simulink model "Laboratoria_nr_6_filtr_SIMULINK"  (R2019a)
settings: Solver=VariableStepAuto  StartTime=0.0  StopTime=2  RelTol=1e-3
libraries: dspsrcs4 x2
settings Model: Creator=mkrup  LastModifiedBy=mkrup

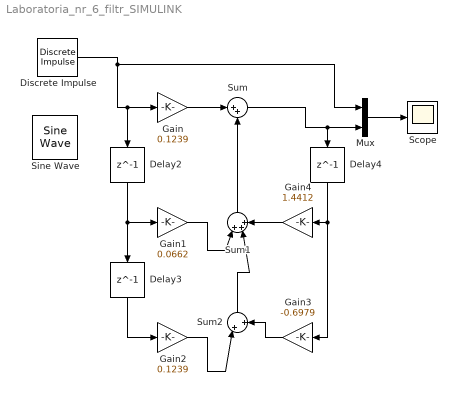
== system Laboratoria_nr_6_filtr_SIMULINK ==
  Delay2 : Delay  DelayLength=1  InitialCondition=0
  Delay3 : Delay  DelayLength=1  InitialCondition=0
  Delay4 : Delay  DelayLength=1  InitialCondition=0
  Discrete Impulse : dspsrcs4/Discrete  Impulse  Delay=10  SampleTime=1/1000  FrameSample=1  OutputFrames=off  dataType=double  isSigned=on  wordLen=16  udDataType=sfix(16)  fracBitsMode=Best precision  numFracBits=15  OutDataTypeStr=double  LastOutDataTypeStr=double
  Gain : Gain  Gain=0.1239
  Gain1 : Gain  Gain=0.0662
  Gain2 : Gain  Gain=0.1239
  Gain3 : Gain  Gain=-0.6979
  Gain4 : Gain  Gain=1.4412
  Mux : Mux  Inputs=2
  Scope : Scope
  Sine Wave : dspsrcs4/Sine Wave  Amplitude=1  Frequency=100  Phase=30  SampleMode=Discrete  OutComplex=Real  CompMethod=Trigonometric fcn  TableSize=Speed  SampleTime=1/1000  SamplesPerFrame=1  ResetState=Restart at time zero  OutputFrames=off  dataType=double  wordLen=16  udDataType=sfix(16)  fracBitsMode=Best precision  numFracBits=15  OutDataTypeStr=double  LastOutDataTypeStr=double
  Sum : Sum  Inputs=|++
  Sum1 : Sum  Inputs=|+++
  Sum2 : Sum  Inputs=|+|+
  wires:
  Gain/1 -> Sum/1
  Sum1/1 -> Sum/2
  Gain1/1 -> Sum1/1
  Gain4/1 -> Sum1/3
  Gain3/1 -> Sum2/2
  Gain2/1 -> Sum2/1
  Mux/1 -> Scope/1
  Sum/1 -> Delay4/1, Mux/2
  Delay2/1 -> Delay3/1, Gain1/1
  Delay3/1 -> Gain2/1
  Delay4/1 -> Gain3/1, Gain4/1
  Sum2/1 -> Sum1/2
  Discrete Impulse/1 -> Mux/1, Delay2/1, Gain/1
